simulink model "example_Hydraulic_Pump"  (R2016b)
settings: Solver=ode45  StartTime=0.0  StopTime=600  RelTol=1e-3  EnableMultiTasking=on
libraries: carnot x8
settings Model: SimulationMode=accelerator  Creator=drhf  LastModifiedBy=drhf
settings DataIOCC: LimitDataPoints=on  SaveFormat=Array  SignalLoggingSaveFormat=ModelDataLogs
settings OptimizationCC: ExpressionDepthLimit=2147483647  LifeSpan=inf
settings DebuggingCC: UnderspecifiedInitializationDetection=Classic  MergeDetectMultiDrivingBlocksExec=none  SolverPrmCheckMsg=warning  FcnCallInpInsideContextMsg=warning  StateNameClashWarn=warning  SFUnexpectedBacktrackingDiag=warning  SFNoUnconditionalDefaultTransitionDiag=warning  SFExecutionAtInitializationDiag=none
settings HardwareCC: ProdBitPerPointer=32  ProdBitPerSizeT=32  ProdBitPerPtrDiffT=32  ProdLargestAtomicFloat=None  ProdIntDivRoundTo=Undefined  ProdEndianess=Unspecified  ProdWordSize=32  ProdHWDeviceType=32-bit Generic
settings ModelReferenceCC: PropagateSignalLabelsOutOfModel=off
settings GRTTargetCC: TargetLangStandard=C89/C90 (ANSI)  GeneratePreprocessorConditionals=Disable all  CombineOutputUpdateFcns=off  GRTInterface=on
settings ConfigComp: CovMetricSettings=dw  CovHtmlReporting=on  CovSaveCumulativeToWorkspaceVar=on  CovSaveSingleToWorkspaceVar=on  CovExternalEMLEnable=off

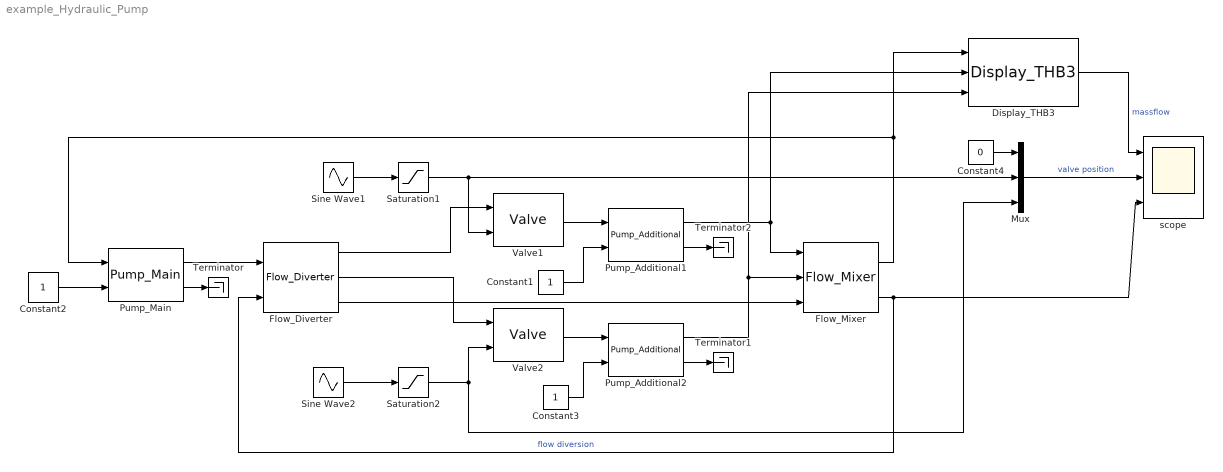
== system example_Hydraulic_Pump ==
  Constant1 : Constant
  Constant2 : Constant
  Constant3 : Constant
  Constant4 : Constant  Value=0
  Display_THB3 : carnot/Outputs/Display_THB3  t=off  m=on  p=off  id=off  mix=off  d=off
  Flow_Diverter : carnot/Hydraulics/Flow_Diverter
  Flow_Mixer : carnot/Hydraulics/Flow_Mixer  t=1
  Mux : Mux  Inputs=3
  Pump_Additional1 : carnot/Hydraulics/Pump_Additional  a0=2.0e4  a1=-7000  a2=0 %-3e-3  dia=0.025  t1=1  ua=0  mcp=0  tamb=0
  Pump_Additional2 : carnot/Hydraulics/Pump_Additional  a0=2.0e4  a1=-7000  a2=0 %-3e-3  dia=0.025  t1=1  ua=0  mcp=0  tamb=0
  Pump_Main : carnot/Hydraulics/Pump_Main  a0=2.7e4  a1=-1.2e4  a2=0%-3e-3  dia=0.025  t1=1  p0=3e5  IDchk=off  fluid_id=Water  mix=0  ua=1  mcp=500  tamb=20
  Saturation1 : Saturate  UpperLimit=1  LowerLimit=0
  Saturation2 : Saturate  UpperLimit=1  LowerLimit=0
  Sine Wave1 : Sin  Amplitude=0.8  Bias=0.5  Frequency=1/60  SampleTime=0
  Sine Wave2 : Sin  Amplitude=0.8  Bias=0.5  Frequency=1/60  Phase=pi  SampleTime=0
  Terminator : Terminator
  Terminator1 : Terminator
  Terminator2 : Terminator
  Valve1 : carnot/Hydraulics/Valve  pos_values=[0 0.1 1]  dp_values=[1e6 1e6 100]
  Valve2 : carnot/Hydraulics/Valve  pos_values=[0 0.1 1]  dp_values=[1e6 1e6 100]
  scope : Scope  NumInputPorts=3
  wires:
  Constant2/1 -> Pump_Main/2
  Pump_Main/2 -> Terminator/1
  Sine Wave1/1 -> Saturation1/1
  Pump_Main/1 -> Flow_Diverter/1
  Flow_Diverter/1 -> Valve1/1
  Sine Wave2/1 -> Saturation2/1
  Flow_Diverter/2 -> Valve2/1
  Flow_Diverter/3 -> Flow_Mixer/3
  Flow_Mixer/2 -> Flow_Diverter/2, scope/3  "flow diversion"
  Flow_Mixer/1 -> Pump_Main/1, Display_THB3/1
  Display_THB3/1 -> scope/1  "massflow"
  Mux/1 -> scope/2  "valve position"
  Valve2/1 -> Pump_Additional2/1
  Pump_Additional2/1 -> Flow_Mixer/2, Display_THB3/3
  Pump_Additional2/2 -> Terminator1/1
  Constant3/1 -> Pump_Additional2/2
  Valve1/1 -> Pump_Additional1/1
  Constant1/1 -> Pump_Additional1/2
  Pump_Additional1/1 -> Flow_Mixer/1, Display_THB3/2
  Pump_Additional1/2 -> Terminator2/1
  Saturation2/1 -> Mux/3, Valve2/2
  Saturation1/1 -> Mux/2, Valve1/2
  Constant4/1 -> Mux/1
